simulink model "WaterSafe"  (R2021b)
settings: Solver=FixedStepAuto  StartTime=0.0  StopTime=sim_time  FixedStep=sim_step  RelTol=1e-3
values from neighbouring files (symbols this model uses):
  A1 = pi*(36/2)^2    (= 1017.87601976)    [simulate_model.m]
  A2 = pi*(36/2)^2    (= 1017.87601976)    [simulate_model.m]
  A3 = pi*(36/2)^2    (= 1017.87601976)    [simulate_model.m]
  A4 = pi*(36/2)^2    (= 1017.87601976)    [simulate_model.m]
  a_1 = 0.107    [simulate_model.m]
  a_2 = 0.107    [simulate_model.m]
  a_3 = 0.107    [simulate_model.m]
  a_4 = 0.107    [simulate_model.m]
  b_1 = 26.59    [simulate_model.m]
  b_2 = 26.59    [simulate_model.m]
  b_3 = 26.59    [simulate_model.m]
  b_4 = 26.59    [simulate_model.m]
  c_1 = -0.97    [simulate_model.m]
  c_2 = -0.97    [simulate_model.m]
  c_3 = -0.97    [simulate_model.m]
  c_4 = -0.97    [simulate_model.m]
  g = 9.80    (= 9.8)    [simulate_model.m]
  gamma_1 = 2.5    [simulate_model.m]
  gamma_2 = 2.5    [simulate_model.m]
  gamma_3 = 2    [simulate_model.m]
  gamma_4 = 2    [simulate_model.m]
  h10 = 21    [simulate_model.m]
  h20 = 20    [simulate_model.m]
  h30 = 17    [simulate_model.m]
  h40 = 19    [simulate_model.m]
  q10 = 0    [simulate_model.m]
  q20 = 0    [simulate_model.m]
  q30 = 0    [simulate_model.m]
  q40 = 0    [simulate_model.m]
  Rl_1 = 20    [simulate_model.m]
  Rl_2 = 16    [simulate_model.m]
  Rl_3 = 16    [simulate_model.m]
  Rl_4 = 15.7    [simulate_model.m]
  Ru_1 = 30    [simulate_model.m]
  Ru_2 = 30    [simulate_model.m]
  Ru_3 = 22    [simulate_model.m]
  Ru_4 = 22.5    [simulate_model.m]
  sim_step = 1    [simulate_model.m]
  t_a_1_1 = 5500    [simulate_model.m]
  t_a_1_2 = 6300    [simulate_model.m]
  t_a_2_1 = 1000    [simulate_model.m]
  t_a_2_2 = 2000    [simulate_model.m]
  t_a_3_1 = 1000    [simulate_model.m]
  t_a_3_2 = 2000    [simulate_model.m]
  t_a_4_1 = 1000    [simulate_model.m]
  t_a_4_2 = 2000    [simulate_model.m]
  t_p_1_1 = 4000    [simulate_model.m]
  t_p_1_2 = 5000    [simulate_model.m]
  t_p_2_1 = 2000    [simulate_model.m]
  t_p_2_2 = 3000    [simulate_model.m]
  t_p_3_1 = 2000    [simulate_model.m]
  t_p_3_2 = 3000    [simulate_model.m]
  t_p_4_1 = 2000    [simulate_model.m]
  t_p_4_2 = 3000    [simulate_model.m]
  t_s_1_1 = 1000    [simulate_model.m]
  t_s_1_2 = 2000    [simulate_model.m]
  t_s_2_1 = 2000    [simulate_model.m]
  t_s_2_2 = 3000    [simulate_model.m]
  t_s_3_1 = 2000    [simulate_model.m]
  t_s_3_2 = 3000    [simulate_model.m]
  t_s_4_1 = 2000    [simulate_model.m]
  t_s_4_2 = 3000    [simulate_model.m]
  theta_a_1 = 0.0    (= 0)    [simulate_model.m]
  theta_a_2 = 0    [simulate_model.m]
  theta_a_3 = 0    [simulate_model.m]
  theta_a_4 = 0    [simulate_model.m]
  theta_p_1 = 0.0    (= 0)    [simulate_model.m]
  theta_p_2 = 0    [simulate_model.m]
  theta_p_3 = 0.0    (= 0)    [simulate_model.m]
  theta_p_4 = 0    [simulate_model.m]
  theta_s_1 = 0    [simulate_model.m]
  theta_s_1_2 = 0.0    (= 0)    [simulate_model.m]
  theta_s_2 = 0    [simulate_model.m]
  theta_s_2_2 = 0    [simulate_model.m]
  theta_s_3 = 0    [simulate_model.m]
  theta_s_3_2 = 0    [simulate_model.m]
  theta_s_4 = 0    [simulate_model.m]
  theta_s_4_2 = 0    [simulate_model.m]
libraries: simulink x8, spsOnDelayLib x4
settings Model: Creator=santr  LastModifiedBy=svrach01
settings SolverCC: AlgebraicLoopSolver=TrustRegion

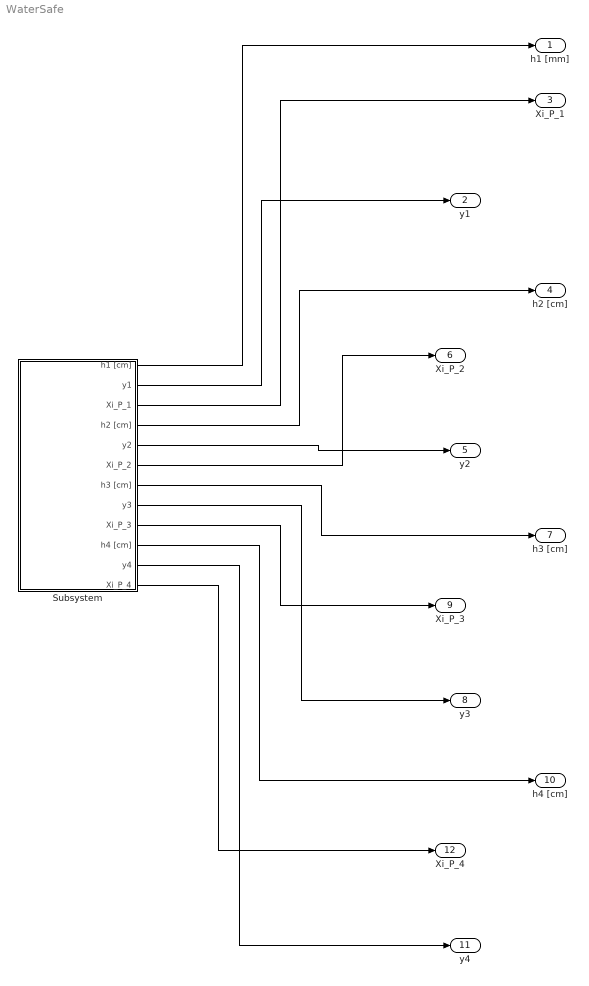
== system WaterSafe ==
  Subsystem : Subsystem
  h1 [mm] : Outport
  y1 : Outport  Port=2
  Xi_P_1 : Outport  Port=3
  h2 [cm] : Outport  Port=4
  y2 : Outport  Port=5
  Xi_P_2 : Outport  Port=6
  h3 [cm] : Outport  Port=7
  y3 : Outport  Port=8
  Xi_P_3 : Outport  Port=9
  h4 [cm] : Outport  Port=10
  y4 : Outport  Port=11
  Xi_P_4 : Outport  Port=12
  wires:
  Subsystem/1(h1 [cm]) -> h1 [mm]/1
  Subsystem/2(y1) -> y1/1
  Subsystem/3(Xi_P_1) -> Xi_P_1/1
  Subsystem/4(h2 [cm]) -> h2 [cm]/1
  Subsystem/5(y2) -> y2/1
  Subsystem/6(Xi_P_2) -> Xi_P_2/1
  Subsystem/7(h3 [cm]) -> h3 [cm]/1
  Subsystem/8(y3) -> y3/1
  Subsystem/9(Xi_P_3) -> Xi_P_3/1
  Subsystem/10(h4 [cm]) -> h4 [cm]/1
  Subsystem/11(y4) -> y4/1
  Subsystem/12(Xi_P_4) -> Xi_P_4/1

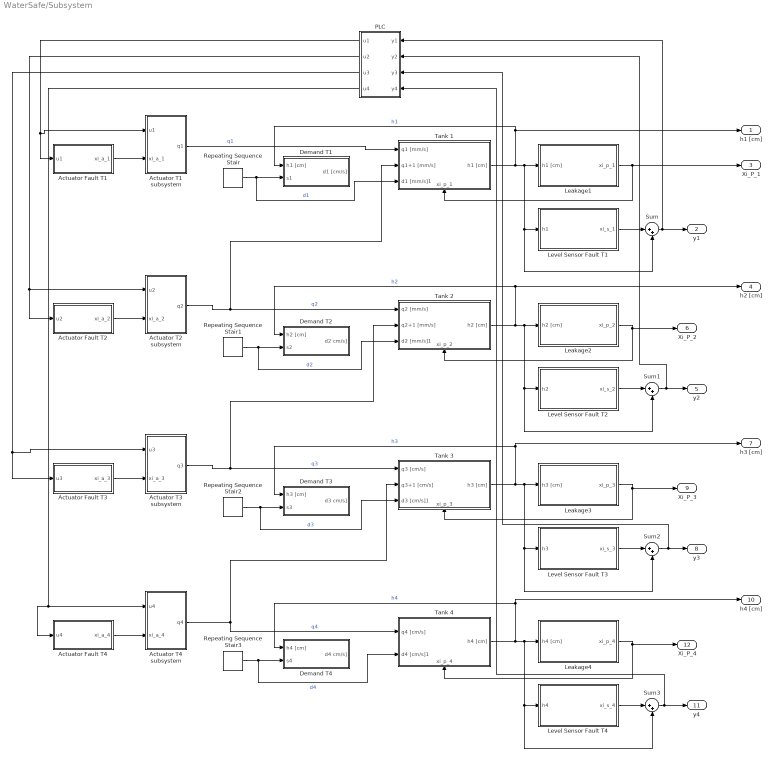
== system WaterSafe/Subsystem ==
  Actuator Fault T1 : Subsystem
  Actuator Fault T2 : Subsystem
  Actuator Fault T3 : Subsystem
  Actuator Fault T4 : Subsystem
  Actuator T1 subsystem : Subsystem
  Actuator T2 subsystem : Subsystem
  Actuator T3 subsystem : Subsystem
  Actuator T4 subsystem : Subsystem
  Demand T1 : Subsystem
  Demand T2 : Subsystem
  Demand T3 : Subsystem
  Demand T4 : Subsystem
  Leakage1 : Subsystem
  Leakage2 : Subsystem
  Leakage3 : Subsystem
  Leakage4 : Subsystem
  Level Sensor Fault T1 : Subsystem
  Level Sensor Fault T2 : Subsystem
  Level Sensor Fault T3 : Subsystem
  Level Sensor Fault T4 : Subsystem
  PLC : Subsystem
  Repeating Sequence Stair : simulink/Sources/Repeating Sequence Stair  OutValues=s1  tsamp=-1  OutMin=[]  OutMax=[]  OutDataTypeStr=double  OutputDataTypeScalingMode=double  OutDataType=fixdt(0,8)  ConRadixGroup=Best Precision: Vector-wise  OutScaling=2^-12
  Repeating Sequence Stair1 : simulink/Sources/Repeating Sequence Stair  OutValues=s2  tsamp=-1  OutMin=[]  OutMax=[]  OutDataTypeStr=double  OutputDataTypeScalingMode=double  OutDataType=fixdt(0,8)  ConRadixGroup=Best Precision: Vector-wise  OutScaling=2^-12
  Repeating Sequence Stair2 : simulink/Sources/Repeating Sequence Stair  OutValues=s3  tsamp=-1  OutMin=[]  OutMax=[]  OutDataTypeStr=double  OutputDataTypeScalingMode=double  OutDataType=fixdt(0,8)  ConRadixGroup=Best Precision: Vector-wise  OutScaling=2^-12
  Repeating Sequence Stair3 : simulink/Sources/Repeating Sequence Stair  OutValues=s4  tsamp=-1  OutMin=[]  OutMax=[]  OutDataTypeStr=double  OutputDataTypeScalingMode=double  OutDataType=fixdt(0,8)  ConRadixGroup=Best Precision: Vector-wise  OutScaling=2^-12
  Sum{,1..3} (4 alike) : Sum  Inputs=|++
  Tank 1 : Subsystem
      settings: PortSchema="{\"entries\":[{\"content\":{\"sides\":[{\"content\":{\"connectorIds\":[\"In1\",\"In2\",\"In3\"]},\"type\":\"ConnectorPlacement.EquallySpacedRectSide\",\"uuid\":\"5502c3df-aac1-47f0-b62d-85524ac4e4b3\"},{\"content\":{\"connectorIds\":[\"Out1\"],\"side\":\"RIGHT\"},\"type\":\"ConnectorPlacement.EquallySpacedRectSide\",\"uuid\":\"388696b2-fbed-4552-a760-e42c088d7a5e\"},{\"content\":{\"connectorIds\":[],\"side\":\"TOP\"},\"type\":\"ConnectorPlacement.EquallySpacedRectSide\",\"uuid\":\"4805e3e6-0573-4070-bd90-a21773e84b57\"},{\"content\":{\"connectorIds\":[\"In4\"],\"side\":\"BOTTOM\"},\"type\":\"ConnectorPlacement.EquallySpacedRectSide\",\"uuid\":\"085ca582-9017-400a-91f9-c572b577085c\"}]},\"type\":\"ConnectorPlacement.EquallySpacedConnector\",\"uuid\":\"4c551cdd-f889-437b-be2d-c0b084ede9dd\"}],\"packageUris\":[\"http://schema.mathworks.com/mf0/Connector/R2020b\"],\"version\":\"1.0\"}"
  Tank 2 : Subsystem
      settings: PortSchema="{\"entries\":[{\"content\":{\"sides\":[{\"content\":{\"connectorIds\":[\"In1\",\"In2\",\"In3\"]},\"type\":\"ConnectorPlacement.EquallySpacedRectSide\",\"uuid\":\"5502c3df-aac1-47f0-b62d-85524ac4e4b3\"},{\"content\":{\"connectorIds\":[\"Out1\"],\"side\":\"RIGHT\"},\"type\":\"ConnectorPlacement.EquallySpacedRectSide\",\"uuid\":\"388696b2-fbed-4552-a760-e42c088d7a5e\"},{\"content\":{\"connectorIds\":[],\"side\":\"TOP\"},\"type\":\"ConnectorPlacement.EquallySpacedRectSide\",\"uuid\":\"4805e3e6-0573-4070-bd90-a21773e84b57\"},{\"content\":{\"connectorIds\":[\"In4\"],\"side\":\"BOTTOM\"},\"type\":\"ConnectorPlacement.EquallySpacedRectSide\",\"uuid\":\"085ca582-9017-400a-91f9-c572b577085c\"}]},\"type\":\"ConnectorPlacement.EquallySpacedConnector\",\"uuid\":\"4c551cdd-f889-437b-be2d-c0b084ede9dd\"}],\"packageUris\":[\"http://schema.mathworks.com/mf0/Connector/R2020b\"],\"version\":\"1.0\"}"
  Tank 3 : Subsystem
      settings: PortSchema="{\"entries\":[{\"content\":{\"sides\":[{\"content\":{\"connectorIds\":[\"In1\",\"In2\",\"In3\"]},\"type\":\"ConnectorPlacement.EquallySpacedRectSide\",\"uuid\":\"5502c3df-aac1-47f0-b62d-85524ac4e4b3\"},{\"content\":{\"connectorIds\":[\"Out1\"],\"side\":\"RIGHT\"},\"type\":\"ConnectorPlacement.EquallySpacedRectSide\",\"uuid\":\"388696b2-fbed-4552-a760-e42c088d7a5e\"},{\"content\":{\"connectorIds\":[],\"side\":\"TOP\"},\"type\":\"ConnectorPlacement.EquallySpacedRectSide\",\"uuid\":\"4805e3e6-0573-4070-bd90-a21773e84b57\"},{\"content\":{\"connectorIds\":[\"In4\"],\"side\":\"BOTTOM\"},\"type\":\"ConnectorPlacement.EquallySpacedRectSide\",\"uuid\":\"085ca582-9017-400a-91f9-c572b577085c\"}]},\"type\":\"ConnectorPlacement.EquallySpacedConnector\",\"uuid\":\"4c551cdd-f889-437b-be2d-c0b084ede9dd\"}],\"packageUris\":[\"http://schema.mathworks.com/mf0/Connector/R2020b\"],\"version\":\"1.0\"}"
  Tank 4 : Subsystem
      settings: PortSchema="{\"entries\":[{\"content\":{\"sides\":[{\"content\":{\"connectorIds\":[\"In1\",\"In2\"]},\"type\":\"ConnectorPlacement.EquallySpacedRectSide\",\"uuid\":\"5502c3df-aac1-47f0-b62d-85524ac4e4b3\"},{\"content\":{\"connectorIds\":[\"Out1\"],\"side\":\"RIGHT\"},\"type\":\"ConnectorPlacement.EquallySpacedRectSide\",\"uuid\":\"388696b2-fbed-4552-a760-e42c088d7a5e\"},{\"content\":{\"connectorIds\":[],\"side\":\"TOP\"},\"type\":\"ConnectorPlacement.EquallySpacedRectSide\",\"uuid\":\"4805e3e6-0573-4070-bd90-a21773e84b57\"},{\"content\":{\"connectorIds\":[\"In3\"],\"side\":\"BOTTOM\"},\"type\":\"ConnectorPlacement.EquallySpacedRectSide\",\"uuid\":\"085ca582-9017-400a-91f9-c572b577085c\"}]},\"type\":\"ConnectorPlacement.EquallySpacedConnector\",\"uuid\":\"4c551cdd-f889-437b-be2d-c0b084ede9dd\"}],\"packageUris\":[\"http://schema.mathworks.com/mf0/Connector/R2020b\"],\"version\":\"1.0\"}"
  h1 [cm] : Outport
  y1 : Outport  Port=2
  Xi_P_1 : Outport  Port=3
  h2 [cm] : Outport  Port=4
  y2 : Outport  Port=5
  Xi_P_2 : Outport  Port=6
  h3 [cm] : Outport  Port=7
  y3 : Outport  Port=8
  Xi_P_3 : Outport  Port=9
  h4 [cm] : Outport  Port=10
  y4 : Outport  Port=11
  Xi_P_4 : Outport  Port=12
  wires:
  Tank 4/1(h4 [cm]) -> Sum3/2, Level Sensor Fault T4/1(h4), Leakage4/1(h4 [cm]), h4 [cm]/1, Demand T4/1(h4 [cm])  "h4"
  PLC/3(u3) -> Actuator T3 subsystem/1(u3), Actuator Fault T3/1(u3)
  Actuator T4 subsystem/1(q4) -> Tank 4/1(q4 [cm/s]), Tank 3/2(q3+1 [cm/s])  "q4"
  Actuator Fault T4/1(xi_a_4) -> Actuator T4 subsystem/2(xi_a_4)
  Sum1/1 -> y2/1, PLC/2(y2)
  Leakage3/1(xi_p_3) -> Xi_P_3/1, Tank 3/4(xi_p_3)
  Repeating Sequence Stair3/1 -> Tank 4/2(d4 [cm/s]1), Demand T4/2(s4)  "d4"
  Leakage4/1(xi_p_4) -> Xi_P_4/1, Tank 4/3(xi_p_4)
  Actuator T3 subsystem/1(q3) -> Tank 2/2(q2+1 [mm/s]), Tank 3/1(q3 [cm/s])  "q3"
  Actuator T2 subsystem/1(q2) -> Tank 1/2(q1+1 [mm/s]), Tank 2/1(q2 [mm/s])  "q2"
  PLC/4(u4) -> Actuator Fault T4/1(u4), Actuator T4 subsystem/1(u4)
  Level Sensor Fault T4/1(xi_s_4) -> Sum3/1
  Level Sensor Fault T3/1(xi_s_3) -> Sum2/1
  Tank 1/1(h1 [cm]) -> Sum/2, Level Sensor Fault T1/1(h1), Leakage1/1(h1 [cm]), h1 [cm]/1, Demand T1/1(h1 [cm])  "h1"
  Actuator Fault T3/1(xi_a_3) -> Actuator T3 subsystem/2(xi_a_3)
  Level Sensor Fault T2/1(xi_s_2) -> Sum1/1
  Actuator Fault T2/1(xi_a_2) -> Actuator T2 subsystem/2(xi_a_2)
  Tank 3/1(h3 [cm]) -> Sum2/2, Level Sensor Fault T3/1(h3), Leakage3/1(h3 [cm]), h3 [cm]/1, Demand T3/1(h3 [cm])  "h3"
  Sum3/1 -> y4/1, PLC/4(y4)
  Repeating Sequence Stair1/1 -> Tank 2/3(d2 [mm/s]1), Demand T2/2(s2)  "d2"
  Leakage1/1(xi_p_1) -> Xi_P_1/1, Tank 1/4(xi_p_1)
  Repeating Sequence Stair/1 -> Tank 1/3(d1 [mm/s]1), Demand T1/2(s1)  "d1"
  Leakage2/1(xi_p_2) -> Xi_P_2/1, Tank 2/4(xi_p_2)
  Sum/1 -> y1/1, PLC/1(y1)
  Actuator Fault T1/1(xi_a_1) -> Actuator T1 subsystem/2(xi_a_1)
  Tank 2/1(h2 [cm]) -> Sum1/2, Level Sensor Fault T2/1(h2), Leakage2/1(h2 [cm]), h2 [cm]/1, Demand T2/1(h2 [cm])  "h2"
  PLC/1(u1) -> Actuator Fault T1/1(u1), Actuator T1 subsystem/1(u1)
  Level Sensor Fault T1/1(xi_s_1) -> Sum/1
  Actuator T1 subsystem/1(q1) -> Tank 1/1(q1 [mm/s])  "q1"
  Repeating Sequence Stair2/1 -> Tank 3/3(d3 [cm/s]1), Demand T3/2(s3)  "d3"
  Sum2/1 -> y3/1, PLC/3(y3)
  PLC/2(u2) -> Actuator Fault T2/1(u2), Actuator T2 subsystem/1(u2)

== system WaterSafe/Subsystem/Actuator Fault T1 ==
  u1 : Inport
  Gain1 : Gain  Gain=theta_a_1
  Product : Product
  Pulse Generator : DiscretePulseGenerator  PulseType=Time based  Amplitude=2  Period=[t_a_1_1, t_a_1_2]
  xi_a_1 : Outport
  wires:
  Product/1 -> xi_a_1/1
  Pulse Generator/1 -> Product/1
  u1/1 -> Gain1/1
  Gain1/1 -> Product/2

== system WaterSafe/Subsystem/Actuator Fault T2 ==
  u2 : Inport
  Gain1 : Gain  Gain=theta_a_2
  Product : Product
  Pulse Generator : DiscretePulseGenerator  PulseType=Time based  Amplitude=0  Period=[t_a_2_1, t_a_2_2]
  xi_a_2 : Outport
  wires:
  Product/1 -> xi_a_2/1
  Pulse Generator/1 -> Product/1
  u2/1 -> Gain1/1
  Gain1/1 -> Product/2

== system WaterSafe/Subsystem/Actuator Fault T3 ==
  u3 : Inport
  Gain1 : Gain  Gain=theta_a_3
  Product : Product
  Pulse Generator : DiscretePulseGenerator  PulseType=Time based  Period=[t_a_3_1, t_a_3_2]
  xi_a_3 : Outport
  wires:
  Product/1 -> xi_a_3/1
  Pulse Generator/1 -> Product/1
  u3/1 -> Gain1/1
  Gain1/1 -> Product/2

== system WaterSafe/Subsystem/Actuator Fault T4 ==
  u4 : Inport
  Gain1 : Gain  Gain=theta_a_4
  Product : Product
  Pulse Generator : DiscretePulseGenerator  PulseType=Time based  Amplitude=2  Period=[t_a_4_1, t_a_4_2]
  xi_a_4 : Outport
  wires:
  Product/1 -> xi_a_4/1
  Pulse Generator/1 -> Product/1
  u4/1 -> Gain1/1
  Gain1/1 -> Product/2

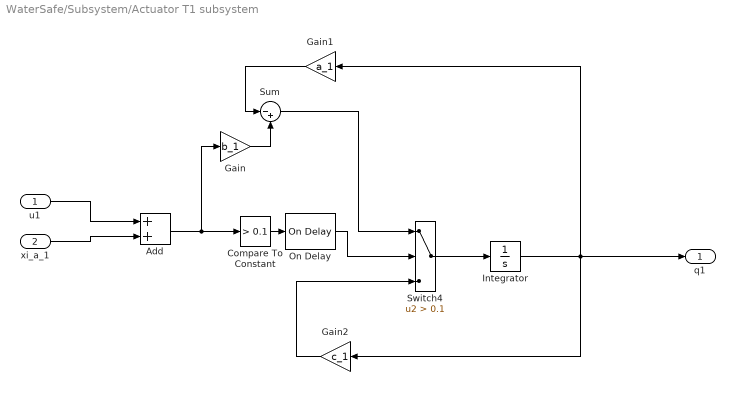
== system WaterSafe/Subsystem/Actuator T1 subsystem ==
  u1 : Inport
  xi_a_1 : Inport  Port=2
  Add : Sum
  Compare To Constant : simulink/Logic and Bit Operations/Compare To Constant  relop=>  const=0.1  OutDataTypeStr=boolean
  Gain : Gain  Gain=b_1
  Gain1 : Gain  Gain=a_1
  Gain2 : Gain  Gain=c_1
  Integrator : Integrator  InitialCondition=q10
  On Delay : spsOnDelayLib/On Delay  DelayType=On delay  delay=20*sim_step  ic=0  Ts=sim_step
      settings: SourceProductBaseCode=PS
  Sum : Sum  Inputs=|-+
  Switch4 : Switch  Criteria=u2 > Threshold  Threshold=0.1
  q1 : Outport
  wires:
  u1/1 -> Add/1
  xi_a_1/1 -> Add/2
  Sum/1 -> Switch4/1
  Gain2/1 -> Switch4/3
  Gain/1 -> Sum/2
  Gain1/1 -> Sum/1
  Add/1 -> Compare To Constant/1, Gain/1
  Switch4/1 -> Integrator/1
  On Delay/1 -> Switch4/2
  Compare To Constant/1 -> On Delay/1
  Integrator/1 -> q1/1, Gain1/1, Gain2/1

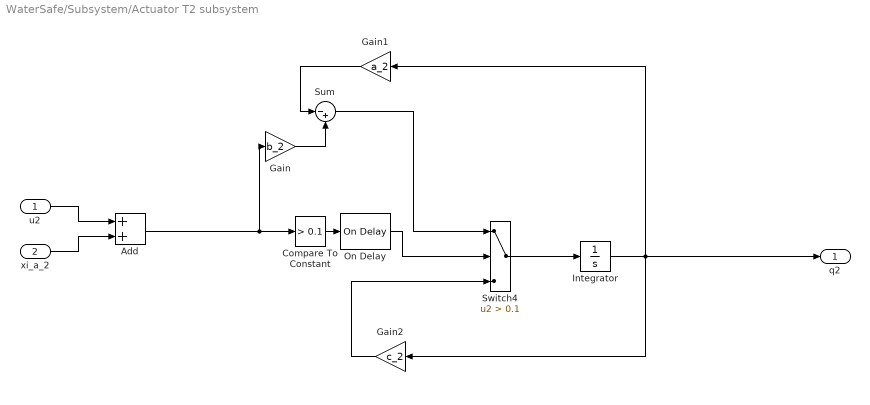
== system WaterSafe/Subsystem/Actuator T2 subsystem ==
  u2 : Inport
  xi_a_2 : Inport  Port=2
  Add : Sum
  Compare To Constant : simulink/Logic and Bit Operations/Compare To Constant  relop=>  const=0.1  OutDataTypeStr=boolean
  Gain : Gain  Gain=b_2
  Gain1 : Gain  Gain=a_2
  Gain2 : Gain  Gain=c_2
  Integrator : Integrator  InitialCondition=q20
  On Delay : spsOnDelayLib/On Delay  DelayType=On delay  delay=20*sim_step  ic=0  Ts=sim_step
      settings: SourceProductBaseCode=PS
  Sum : Sum  Inputs=|-+
  Switch4 : Switch  Criteria=u2 > Threshold  Threshold=0.1
  q2 : Outport
  wires:
  u2/1 -> Add/1
  xi_a_2/1 -> Add/2
  Sum/1 -> Switch4/1
  Gain2/1 -> Switch4/3
  Gain/1 -> Sum/2
  Gain1/1 -> Sum/1
  Add/1 -> Compare To Constant/1, Gain/1
  Switch4/1 -> Integrator/1
  Compare To Constant/1 -> On Delay/1
  On Delay/1 -> Switch4/2
  Integrator/1 -> q2/1, Gain1/1, Gain2/1

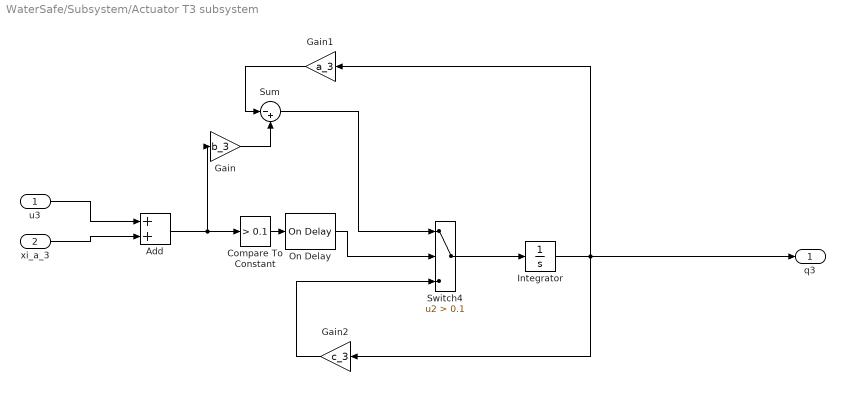
== system WaterSafe/Subsystem/Actuator T3 subsystem ==
  u3 : Inport
  xi_a_3 : Inport  Port=2
  Add : Sum
  Compare To Constant : simulink/Logic and Bit Operations/Compare To Constant  relop=>  const=0.1  OutDataTypeStr=boolean
  Gain : Gain  Gain=b_3
  Gain1 : Gain  Gain=a_3
  Gain2 : Gain  Gain=c_3
  Integrator : Integrator  InitialCondition=q30
  On Delay : spsOnDelayLib/On Delay  DelayType=On delay  delay=20*sim_step  ic=0  Ts=sim_step
      settings: SourceProductBaseCode=PS
  Sum : Sum  Inputs=|-+
  Switch4 : Switch  Criteria=u2 > Threshold  Threshold=0.1
  q3 : Outport
  wires:
  u3/1 -> Add/1
  xi_a_3/1 -> Add/2
  Sum/1 -> Switch4/1
  Gain2/1 -> Switch4/3
  Gain/1 -> Sum/2
  Gain1/1 -> Sum/1
  Add/1 -> Compare To Constant/1, Gain/1
  Switch4/1 -> Integrator/1
  On Delay/1 -> Switch4/2
  Compare To Constant/1 -> On Delay/1
  Integrator/1 -> q3/1, Gain1/1, Gain2/1

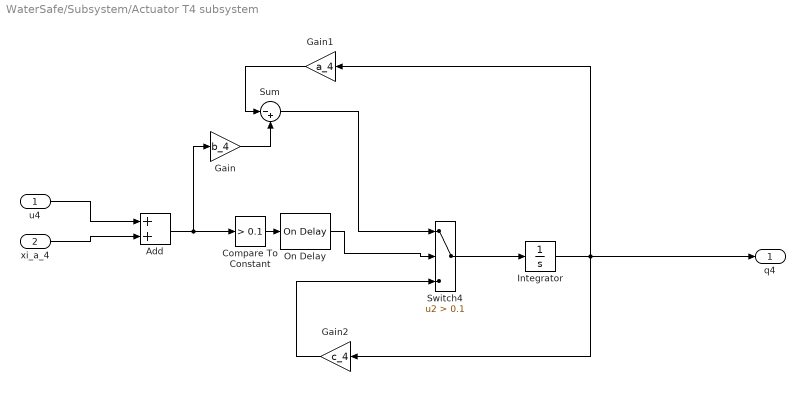
== system WaterSafe/Subsystem/Actuator T4 subsystem ==
  u4 : Inport
  xi_a_4 : Inport  Port=2
  Add : Sum
  Compare To Constant : simulink/Logic and Bit Operations/Compare To Constant  relop=>  const=0.1  OutDataTypeStr=boolean
  Gain : Gain  Gain=b_4
  Gain1 : Gain  Gain=a_4
  Gain2 : Gain  Gain=c_4
  Integrator : Integrator  InitialCondition=q40
  On Delay : spsOnDelayLib/On Delay  DelayType=On delay  delay=20*sim_step  ic=0  Ts=sim_step
      settings: SourceProductBaseCode=PS
  Sum : Sum  Inputs=|-+
  Switch4 : Switch  Criteria=u2 > Threshold  Threshold=0.1
  q4 : Outport
  wires:
  u4/1 -> Add/1
  xi_a_4/1 -> Add/2
  Sum/1 -> Switch4/1
  Gain2/1 -> Switch4/3
  Gain/1 -> Sum/2
  Gain1/1 -> Sum/1
  Add/1 -> Compare To Constant/1, Gain/1
  Switch4/1 -> Integrator/1
  Compare To Constant/1 -> On Delay/1
  On Delay/1 -> Switch4/2
  Integrator/1 -> q4/1, Gain1/1, Gain2/1

== system WaterSafe/Subsystem/Demand T1 ==
  h1 [cm] : Inport
  s1 : Inport  Port=2
  Gain : Gain  Gain=gamma_1
  Gain1 : Gain  Gain=2*g
  Product1 : Product
  Sqrt : Sqrt  SaturateOnIntegerOverflow=on
  d1 [cm/s] : Outport
  wires:
  Sqrt/1 -> Product1/1
  Gain1/1 -> Sqrt/1
  h1 [cm]/1 -> Gain1/1
  Product1/1 -> d1 [cm/s]/1
  s1/1 -> Gain/1
  Gain/1 -> Product1/2

== system WaterSafe/Subsystem/Demand T2 ==
  h2 [cm] : Inport
  s2 : Inport  Port=2
  Gain : Gain  Gain=gamma_2
  Gain1 : Gain  Gain=2*g
  Product1 : Product
  Sqrt : Sqrt  SaturateOnIntegerOverflow=on
  d2 cm/s] : Outport
  wires:
  Sqrt/1 -> Product1/1
  Gain1/1 -> Sqrt/1
  h2 [cm]/1 -> Gain1/1
  Product1/1 -> d2 cm/s]/1
  s2/1 -> Gain/1
  Gain/1 -> Product1/2

== system WaterSafe/Subsystem/Demand T3 ==
  h3 [cm] : Inport
  s3 : Inport  Port=2
  Gain : Gain  Gain=gamma_3
  Gain1 : Gain  Gain=2*g
  Product1 : Product
  Sqrt : Sqrt  SaturateOnIntegerOverflow=on
  d3 cm/s] : Outport
  wires:
  Sqrt/1 -> Product1/1
  Gain1/1 -> Sqrt/1
  h3 [cm]/1 -> Gain1/1
  Product1/1 -> d3 cm/s]/1
  s3/1 -> Gain/1
  Gain/1 -> Product1/2

== system WaterSafe/Subsystem/Demand T4 ==
  h4 [cm] : Inport
  s4 : Inport  Port=2
  Gain : Gain  Gain=gamma_4
  Gain1 : Gain  Gain=2*g
  Product1 : Product
  Sqrt : Sqrt  SaturateOnIntegerOverflow=on
  d4 cm/s] : Outport
  wires:
  Sqrt/1 -> Product1/1
  Gain1/1 -> Sqrt/1
  h4 [cm]/1 -> Gain1/1
  Product1/1 -> d4 cm/s]/1
  s4/1 -> Gain/1
  Gain/1 -> Product1/2

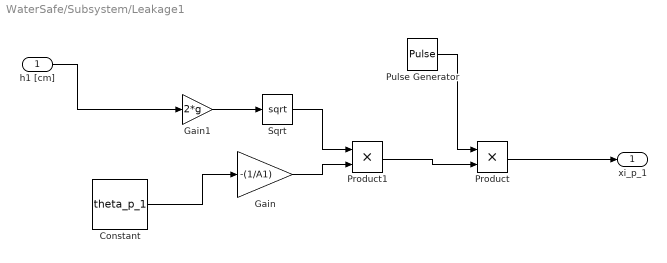
== system WaterSafe/Subsystem/Leakage1 ==
  h1 [cm] : Inport
  Constant : Constant  Value=theta_p_1
  Gain : Gain  Gain=-(1/A1)
  Gain1 : Gain  Gain=2*g
  Product : Product
  Product1 : Product
  Pulse Generator : DiscretePulseGenerator  PulseType=Time based  Amplitude=4  Period=[t_p_1_1, t_p_1_2]  PulseWidth=5
  Sqrt : Sqrt  SaturateOnIntegerOverflow=on
  xi_p_1 : Outport
  wires:
  Product/1 -> xi_p_1/1
  Pulse Generator/1 -> Product/1
  Product1/1 -> Product/2
  Gain1/1 -> Sqrt/1
  Sqrt/1 -> Product1/1
  h1 [cm]/1 -> Gain1/1
  Gain/1 -> Product1/2
  Constant/1 -> Gain/1

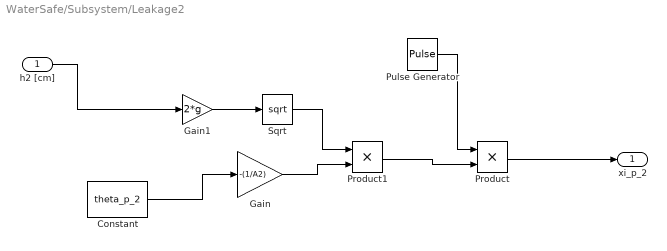
== system WaterSafe/Subsystem/Leakage2 ==
  h2 [cm] : Inport
  Constant : Constant  Value=theta_p_2
  Gain : Gain  Gain=-(1/A2)
  Gain1 : Gain  Gain=2*g
  Product : Product
  Product1 : Product
  Pulse Generator : DiscretePulseGenerator  PulseType=Time based  Amplitude=4  Period=[t_p_2_1, t_p_2_2]  PulseWidth=5
  Sqrt : Sqrt  SaturateOnIntegerOverflow=on
  xi_p_2 : Outport
  wires:
  Product/1 -> xi_p_2/1
  Pulse Generator/1 -> Product/1
  Product1/1 -> Product/2
  Gain1/1 -> Sqrt/1
  Sqrt/1 -> Product1/1
  h2 [cm]/1 -> Gain1/1
  Gain/1 -> Product1/2
  Constant/1 -> Gain/1

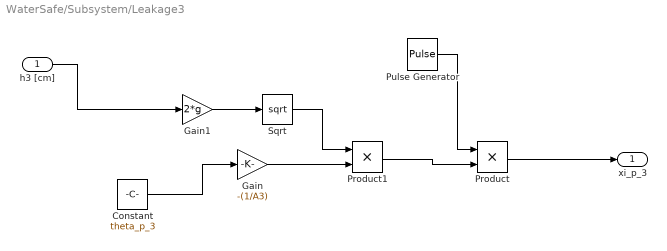
== system WaterSafe/Subsystem/Leakage3 ==
  h3 [cm] : Inport
  Constant : Constant  Value=theta_p_3
  Gain : Gain  Gain=-(1/A3)
  Gain1 : Gain  Gain=2*g
  Product : Product
  Product1 : Product
  Pulse Generator : DiscretePulseGenerator  PulseType=Time based  Amplitude=4  Period=[t_p_3_1, t_p_3_2]  PulseWidth=5
  Sqrt : Sqrt  SaturateOnIntegerOverflow=on
  xi_p_3 : Outport
  wires:
  Product/1 -> xi_p_3/1
  Pulse Generator/1 -> Product/1
  Product1/1 -> Product/2
  Gain1/1 -> Sqrt/1
  Sqrt/1 -> Product1/1
  h3 [cm]/1 -> Gain1/1
  Gain/1 -> Product1/2
  Constant/1 -> Gain/1

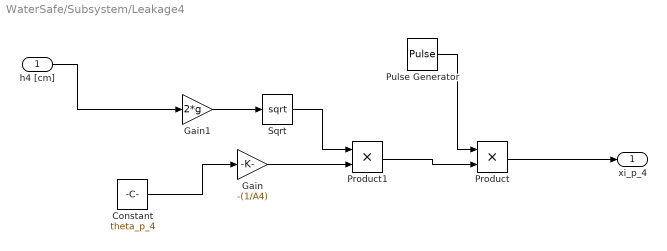
== system WaterSafe/Subsystem/Leakage4 ==
  h4 [cm] : Inport
  Constant : Constant  Value=theta_p_4
  Gain : Gain  Gain=-(1/A4)
  Gain1 : Gain  Gain=2*g
  Product : Product
  Product1 : Product
  Pulse Generator : DiscretePulseGenerator  PulseType=Time based  Amplitude=4  Period=[t_p_4_1, t_p_4_2]  PulseWidth=5
  Sqrt : Sqrt  SaturateOnIntegerOverflow=on
  xi_p_4 : Outport
  wires:
  Product/1 -> xi_p_4/1
  Pulse Generator/1 -> Product/1
  Product1/1 -> Product/2
  Gain1/1 -> Sqrt/1
  Sqrt/1 -> Product1/1
  h4 [cm]/1 -> Gain1/1
  Gain/1 -> Product1/2
  Constant/1 -> Gain/1

== system WaterSafe/Subsystem/Level Sensor Fault T1 ==
  h1 : Inport
  Constant : Constant  Value=theta_s_1_2
  Gain1 : Gain  Gain=theta_s_1
  Product : Product
  Pulse Generator : DiscretePulseGenerator  PulseType=Time based  Amplitude=2  Period=[t_s_1_1, t_s_1_2]  PulseWidth=50
  Sum : Sum  Inputs=|++
  xi_s_1 : Outport
  wires:
  Product/1 -> xi_s_1/1
  Pulse Generator/1 -> Product/1
  h1/1 -> Gain1/1
  Sum/1 -> Product/2
  Gain1/1 -> Sum/1
  Constant/1 -> Sum/2

== system WaterSafe/Subsystem/Level Sensor Fault T2 ==
  h2 : Inport
  Constant : Constant  Value=theta_s_2_2
  Gain1 : Gain  Gain=theta_s_2
  Product : Product
  Pulse Generator : DiscretePulseGenerator  PulseType=Time based  Amplitude=2  Period=[t_s_2_1, t_s_2_2]  PulseWidth=5
  Sum : Sum  Inputs=|++
  xi_s_2 : Outport
  wires:
  Product/1 -> xi_s_2/1
  Pulse Generator/1 -> Product/1
  h2/1 -> Gain1/1
  Sum/1 -> Product/2
  Gain1/1 -> Sum/1
  Constant/1 -> Sum/2

== system WaterSafe/Subsystem/Level Sensor Fault T3 ==
  h3 : Inport
  Constant : Constant  Value=theta_s_3_2
  Gain1 : Gain  Gain=theta_s_3
  Product : Product
  Pulse Generator : DiscretePulseGenerator  PulseType=Time based  Amplitude=2  Period=[t_s_3_1, t_s_3_2]  PulseWidth=5
  Sum : Sum  Inputs=|++
  xi_s_3 : Outport
  wires:
  Product/1 -> xi_s_3/1
  Pulse Generator/1 -> Product/1
  h3/1 -> Gain1/1
  Sum/1 -> Product/2
  Gain1/1 -> Sum/1
  Constant/1 -> Sum/2

== system WaterSafe/Subsystem/Level Sensor Fault T4 ==
  h4 : Inport
  Constant : Constant  Value=theta_s_4_2
  Gain1 : Gain  Gain=theta_s_4
  Product : Product
  Pulse Generator : DiscretePulseGenerator  PulseType=Time based  Amplitude=2  Period=[t_s_4_1, t_s_4_2]  PulseWidth=5
  Sum : Sum  Inputs=|++
  xi_s_4 : Outport
  wires:
  Product/1 -> xi_s_4/1
  Pulse Generator/1 -> Product/1
  h4/1 -> Gain1/1
  Sum/1 -> Product/2
  Gain1/1 -> Sum/1
  Constant/1 -> Sum/2

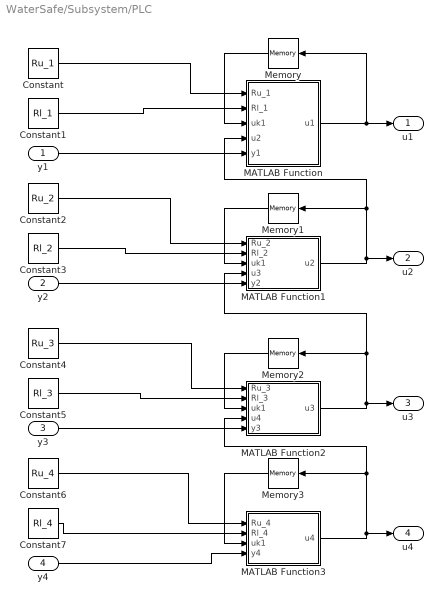
== system WaterSafe/Subsystem/PLC ==
  y1 : Inport
  y2 : Inport  Port=2
  y3 : Inport  Port=3
  y4 : Inport  Port=4
  Constant : Constant  Value=Ru_1
  Constant1 : Constant  Value=Rl_1
  Constant2 : Constant  Value=Ru_2
  Constant3 : Constant  Value=Rl_2
  Constant4 : Constant  Value=Ru_3
  Constant5 : Constant  Value=Rl_3
  Constant6 : Constant  Value=Ru_4
  Constant7 : Constant  Value=Rl_4
  MATLAB Function : MATLAB Function  TreatAsAtomicUnit=on
  MATLAB Function1 : MATLAB Function  TreatAsAtomicUnit=on
  MATLAB Function2 : MATLAB Function  TreatAsAtomicUnit=on
  MATLAB Function3 : MATLAB Function  TreatAsAtomicUnit=on
  Memory{,1..3} (4 alike) : Memory
  u1 : Outport
  u2 : Outport  Port=2
  u3 : Outport  Port=3
  u4 : Outport  Port=4
  wires:
  y1/1 -> MATLAB Function/5(y1)
  MATLAB Function/1(u1) -> Memory/1, u1/1
  Memory/1 -> MATLAB Function/3(uk1)
  Memory1/1 -> MATLAB Function1/3(uk1)
  MATLAB Function1/1(u2) -> MATLAB Function/4(u2), Memory1/1, u2/1
  Memory2/1 -> MATLAB Function2/3(uk1)
  MATLAB Function2/1(u3) -> MATLAB Function1/4(u3), Memory2/1, u3/1
  y3/1 -> MATLAB Function2/5(y3)
  Memory3/1 -> MATLAB Function3/3(uk1)
  MATLAB Function3/1(u4) -> MATLAB Function2/4(u4), Memory3/1, u4/1
  y4/1 -> MATLAB Function3/4(y4)
  Constant/1 -> MATLAB Function/1(Ru_1)
  Constant1/1 -> MATLAB Function/2(Rl_1)
  Constant3/1 -> MATLAB Function1/2(Rl_2)
  Constant2/1 -> MATLAB Function1/1(Ru_2)
  Constant5/1 -> MATLAB Function2/2(Rl_3)
  Constant4/1 -> MATLAB Function2/1(Ru_3)
  Constant7/1 -> MATLAB Function3/2(Rl_4)
  Constant6/1 -> MATLAB Function3/1(Ru_4)
  y2/1 -> MATLAB Function1/5(y2)

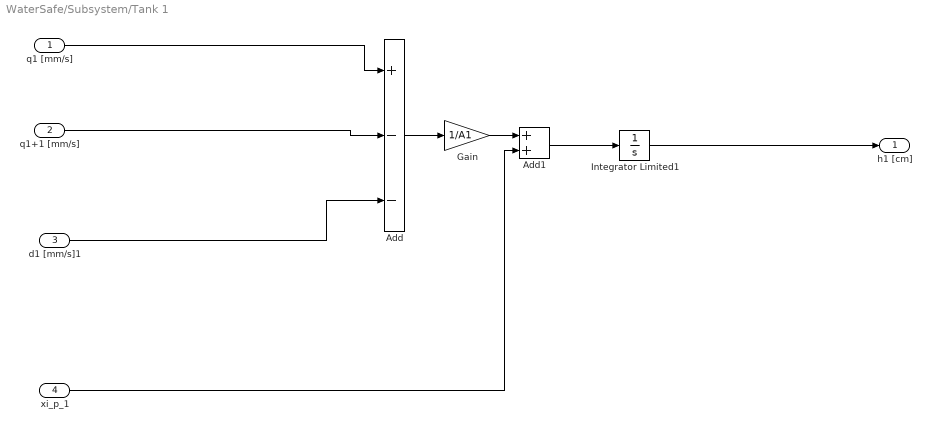
== system WaterSafe/Subsystem/Tank 1 ==
  q1 [mm/s] : Inport
  q1+1 [mm/s] : Inport  Port=2
  d1 [mm/s]1 : Inport  Port=3
  xi_p_1 : Inport  Port=4
  Add : Sum  Inputs=+--
  Add1 : Sum
  Gain : Gain  Gain=1/A1
  Integrator Limited1 : Integrator  InitialCondition=h10  UpperSaturationLimit=270  LowerSaturationLimit=100
  h1 [cm] : Outport
  wires:
  q1 [mm/s]/1 -> Add/1
  d1 [mm/s]1/1 -> Add/3
  q1+1 [mm/s]/1 -> Add/2
  Add/1 -> Gain/1
  Gain/1 -> Add1/1
  Add1/1 -> Integrator Limited1/1
  xi_p_1/1 -> Add1/2
  Integrator Limited1/1 -> h1 [cm]/1

== system WaterSafe/Subsystem/Tank 2 ==
  q2 [mm/s] : Inport
  q2+1 [mm/s] : Inport  Port=2
  d2 [mm/s]1 : Inport  Port=3
  xi_p_2 : Inport  Port=4
  Add : Sum  Inputs=+--
  Add1 : Sum
  Gain : Gain  Gain=1/A2
  Integrator Limited1 : Integrator  InitialCondition=h20  UpperSaturationLimit=270  LowerSaturationLimit=100
  h2 [cm] : Outport
  wires:
  q2 [mm/s]/1 -> Add/1
  d2 [mm/s]1/1 -> Add/3
  q2+1 [mm/s]/1 -> Add/2
  Add/1 -> Gain/1
  Gain/1 -> Add1/1
  Add1/1 -> Integrator Limited1/1
  xi_p_2/1 -> Add1/2
  Integrator Limited1/1 -> h2 [cm]/1

== system WaterSafe/Subsystem/Tank 3 ==
  q3 [cm/s] : Inport
  q3+1 [cm/s] : Inport  Port=2
  d3 [cm/s]1 : Inport  Port=3
  xi_p_3 : Inport  Port=4
  Add : Sum  Inputs=+--
  Add1 : Sum
  Gain : Gain  Gain=1/A3
  Integrator Limited1 : Integrator  InitialCondition=h30  UpperSaturationLimit=270  LowerSaturationLimit=100
  h3 [cm] : Outport
  wires:
  q3 [cm/s]/1 -> Add/1
  d3 [cm/s]1/1 -> Add/3
  q3+1 [cm/s]/1 -> Add/2
  Add/1 -> Gain/1
  Gain/1 -> Add1/1
  Add1/1 -> Integrator Limited1/1
  xi_p_3/1 -> Add1/2
  Integrator Limited1/1 -> h3 [cm]/1

== system WaterSafe/Subsystem/Tank 4 ==
  q4 [cm/s] : Inport
  d4 [cm/s]1 : Inport  Port=2
  xi_p_4 : Inport  Port=3
  Add : Sum  Inputs=+-
  Add1 : Sum
  Gain : Gain  Gain=1/A4
  Integrator Limited1 : Integrator  InitialCondition=h40  UpperSaturationLimit=270  LowerSaturationLimit=100
  h4 [cm] : Outport
  wires:
  q4 [cm/s]/1 -> Add/1
  d4 [cm/s]1/1 -> Add/2
  Add/1 -> Gain/1
  Gain/1 -> Add1/1
  Add1/1 -> Integrator Limited1/1
  xi_p_4/1 -> Add1/2
  Integrator Limited1/1 -> h4 [cm]/1

== matlab function WaterSafe/Subsystem/PLC/MATLAB Function1 ==
  data: Ru_2 input; Rl_2 input; uk1 input; u3 input; u2 output; y2 input
function u2 = fcn(Ru_2,Rl_2,uk1,u3,y2)
% Ru=27;
% Rl=10;
if (min(y2)<=Rl_2 && u3>=0.1)
    u2=0.85;
elseif (min(y2)<=Rl_2 && u3<0.1)
    u2=0.25;
elseif min(y2)>=Ru_2
    u2=0.0;
else
    u2 = uk1;
end

end

== matlab function WaterSafe/Subsystem/PLC/MATLAB Function ==
  data: Ru_1 input; Rl_1 input; uk1 input; u2 input; y1 input; u1 output
function u1 = fcn(Ru_1, Rl_1, uk1, u2, y1)
% Ru=25;
% Rl=10;
if (min(y1)<=Rl_1 & u2>=0.1)
    u1=0.95;
elseif (min(y1)<=Rl_1 & u2<0.1)
    u1=0.47;
elseif min(y1)>=Ru_1
    u1=-0.00;
else
    u1 = uk1;
end

end

== matlab function WaterSafe/Subsystem/PLC/MATLAB Function2 ==
  data: Ru_3 input; Rl_3 input; uk1 input; u4 input; y3 input; u3 output
function u3 = fcn(Ru_3, Rl_3, uk1, u4, y3)
% Ru=27;
% Rl=10;
if (min(y3)<=Rl_3 && u4>=0.1)
    u3=0.55;
elseif (min(y3)<=Rl_3 && u4<0.1)
    u3=0.22;
elseif min(y3)>=Ru_3
    u3=0;
else
    u3 = uk1;
end

end

== matlab function WaterSafe/Subsystem/PLC/MATLAB Function3 ==
  data: Ru_4 input; Rl_4 input; uk1 input; y4 input; u4 output
function u4 = fcn(Ru_4, Rl_4, uk1, y4)
% Ru=27;
% Rl=10;
if y4<=Rl_4
    u4=0.18;
elseif y4>=Ru_4
    u4=0;
else
    u4 = uk1;
end

end
